simulink model "car_sim"  (R2022a)
settings: Solver=FixedStepAuto  StartTime=0.0  StopTime=40  FixedStep=0.001  RelTol=1e-3
InitFcn:
  | init_car_dynamic
StopFcn:
  | plot_traj_results
undefined symbols (not defined in the file or in its folder): ctrl_K, ctrl_K_lqi, ModelParams, my_traj, track, trackWidth, traj, vx
libraries: slpidlib x3
settings Model: Creator=Manny  LastModifiedBy=zqsyx
settings SolverCC: AlgebraicLoopSolver=LineSearch
settings DebuggingCC: UnconnectedInputMsg=warning  UnconnectedOutputMsg=warning  UnconnectedLineMsg=warning  SFMachineParentedDataDiag=warning
settings RTWCC: DLArmComputeVersion=19.05

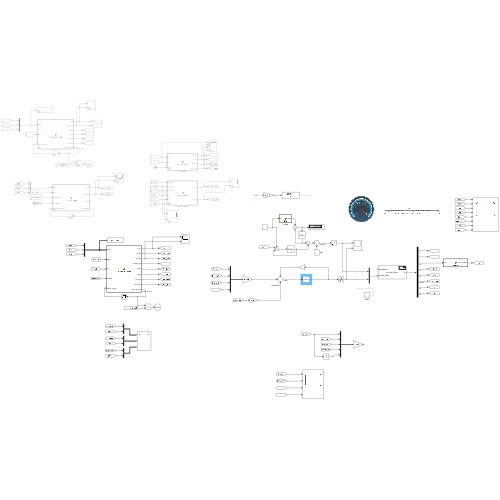
[thumbnail: Simulink's stored preview of the top-level diagram]
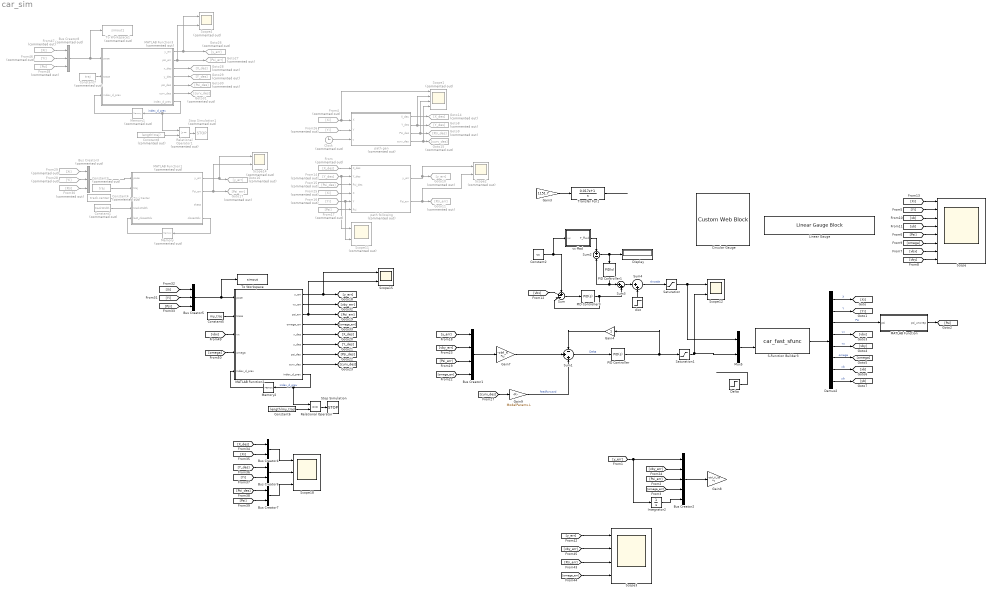
== system car_sim ==
  Bus Creator1 : BusCreator  Inputs=4
  Bus Creator2 : BusCreator  Inputs=5
  Bus Creator3 : BusCreator  Commented=on  Inputs=3
  Bus Creator4 : BusCreator  Inputs=2
  Bus Creator5 : BusCreator  Inputs=3
  Bus Creator6 : BusCreator  Inputs=2
  Bus Creator7 : BusCreator  Inputs=2
  Bus Creator8 : BusCreator  Commented=on  Inputs=3
  Circular Gauge : CustomWebBlock  LabelPosition=Hide  ShowInitialText=on  Configuration="{\"components\":[{\"name\":\"CircularScaleComponent\",\"settings\":{\"bounds\":{\"max\":1,\"min\":0,\"tickInterval\":\"auto\"},\"direction\":\"cw\",\"flipLimits\":0,\"innerRadius\":0.75,\"internalTickHeightScaleFactor\":1,\"labelColor\":[255,252,199],\"labelFont\":{\"font\":\"Arial\",\"fontSize\":12},\"labelTransparency\":1,\"minorTickHeightScaleFactor\":0.2,\"needleImage\":{\"size\":[1890,567],\"src\":\"data:image\\/svg+xml;base64,PD94bWwgdmVyc2lvbj0iMS4wIiBlbmNvZGluZz0iVVRGLTgiIHN0YW5kYWxvbmU9Im5vIj8+CjxzdmcKICAgeG1sbnM6ZGM9Imh0dHA6Ly9wdXJsLm9yZy9kYy9lbGVtZW50cy8xLjEvIgogICB4bWxuczpjYz0iaHR0cDovL2NyZWF0aXZlY29tbW9ucy5vcmcvbnMjIgogICB4bWxuczpyZGY9Imh0dHA6Ly93d3cudzMub3JnLzE5OTkvMDIvMjItcmRmLXN5bnRheC1ucyMiCiAgIHhtbG5zOnN2Zz0iaHR0cDovL3d3dy53My5vcmcvMjAwMC9zdmciCiAgIHhtbG5zPSJodHRwOi8vd3d3LnczLm9yZy8yMDAwL3N2ZyIKICAgeG1sbnM6 ...(+4096 chars)\"},\"needleOffset\":[0.1610917094974375,0],\"needleOrientation\":-45,\"needleRotation\":180.59702388394928,\"needleSize\":{\"height\":0.13032601008944536,\"width\":0.416859542883425},\"outerRadius\":0.9,\"position\":[0.06486742424242424,0.05627705627705628,0.8917748917748918,0.8787878787878788],\"scaleAngle\":270,\"scaleAngleOffset\":135,\"scaleColors\":[{\"color\":[0,114,189],\"max\":0.8,\"min\":0},{\"color\":[217,83,25],\"max\":1,\"min\":0.81}],\"scaleColorsSize\":0.2,\"scalePosition\":[0,0,1,1],\"showLabels\":1,\"showMinorTicks\":1,\"showSpanLine\":1,\"showTicks\":1,\"tickColor\":[255,255,200],\"tickTransparency\":1,\"valueBarColor\":[0,114,189],\"valueBarPosition\":[0,0,1,1],\"valueBarSize\":0.2,\"valueBarTransparency\":1}},{\"name\":\"BackgroundImageComponent\",\"settings\":{\"image\":{\"size\":[500,500],\"src\":\"data:image\\/svg+xml;base64,PD94bWwgdmVyc2lvbj0iMS4wIiBlbmNvZGluZz0iVVRGLTgiIHN0YW5kYWxvbmU9Im5vIj8+CjxzdmcKICAgeG1sbnM6ZGM9Imh0dHA6Ly9wdXJsLm9yZy9kYy9lbGVtZW50cy8xLjEvIgogICB4bWxuczpjYz0iaHR0cDovL2NyZWF0aXZlY29tbW9ucy5vcmcvbnMjIgogICB4bWxuczpyZGY9Imh0dHA6Ly93d3cudzMub3JnLzE5OTkvMDIvMjItcmRmLXN5bnRheC1ucyMiCiAgIHhtbG5zOnN2Zz0iaHR0cDovL3d3dy53My5vcmcvMjAwMC9zdmciCiAgIHhtbG5zPSJodHRwOi8vd3d3LnczLm9yZy8yMDAwL3N2ZyIKICAgeG1sbnM6 ...(+9964 chars)\"},\"position\":[0,0,1,1],\"scaleMode\":\"0\"}},{\"name\":\"ForegroundImageComponent\",\"settings\":{\"image\":{\"size\":[0,0],\"src\":\"default\",\"srcOrientation\":[]},\"isForeground\":1,\"position\":[0,0,1,1],\"scaleMode\":\"0\"}}],\"settings\":{\"BindingType\":\"signal\",\"aspectRatio\":1.0330578512396693,\"direction\":\"cw\",\"fixedAspectRatio\":\"on\",\"flipLimits\":0,\"orientation\":\"horizontal\"},\"type\":\"CircularGauge\"}"
  Clock : Clock  Commented=on
  Constant1 : Constant  Commented=on  Value=trackWidth
  Constant2 : Constant  Value=vx
  Constant3 : Constant  Commented=on  Value=traj  VectorParams1D=off  OutDataTypeStr=Bus: traj_bus
  Constant4 : Constant  Commented=on  Value=track.center
  Constant5 : Constant  Value=my_traj
  Constant6 : Constant  Value=length(my_traj)
  Constant7 : Constant  Commented=on  Value=traj
  Constant8 : Constant  Commented=on  Value=length(traj)
  Delta : Step  Time=5  After=0.05  SampleTime=0
  Demux2 : Demux  Outputs=8
  Display : Display
  From : From  Commented=on  GotoTag=X_des
  From14 : From  Commented=on  GotoTag=Y_des
  From15 : From  Commented=on  GotoTag=Psi_des
  From{16,26,28,46} (4 alike) : From  Commented=on  GotoTag=Yi
  From17 : From  Commented=on  GotoTag=Psi
  From{4,25,29,47} (4 alike) : From  Commented=on  GotoTag=Xi
  From30 : From  Commented=on  GotoTag=Psi
  From48 : From  Commented=on  GotoTag=Psi
  Gain3 : Gain  Gain=1151.7
  Gain4 : Gain
  Gain7 : Gain  Gain=-ctrl_K  Multiplication=Matrix(K*u) (u vector)
  Gain8 : Gain  Gain=-ctrl_K_lqi  Multiplication=Matrix(K*u) (u vector)
  Gain9 : Gain  Gain=ModelParams.L
  Goto10 : Goto  Commented=on  GotoTag=y_err
  Goto11 : Goto  Commented=on  GotoTag=Psi_err
  Goto14 : Goto  Commented=on  GotoTag=X_des
  Goto15 : Goto  Commented=on  GotoTag=curv_des
  Goto16 : Goto  Commented=on  GotoTag=y_err
  Goto17 : Goto  Commented=on  GotoTag=Psi_err
  Goto26 : Goto  Commented=on  GotoTag=y_err
  Goto27 : Goto  Commented=on  GotoTag=Psi_err
  Goto28 : Goto  Commented=on  GotoTag=X_des
  Goto29 : Goto  Commented=on  GotoTag=Y_des
  Goto30 : Goto  Commented=on  GotoTag=Psi_des
  Goto31 : Goto  Commented=on  GotoTag=curv_des
  Goto8 : Goto  Commented=on  GotoTag=Y_des
  Goto9 : Goto  Commented=on  GotoTag=Psi_des
  Integrator2 : Integrator
  Linear Gauge : LinearGaugeBlock  ScaleMin=-1.5  ScaleMax=1.5
  MATLAB Function : MATLAB Function  TreatAsAtomicUnit=on
  MATLAB Function1 : MATLAB Function  Commented=on  TreatAsAtomicUnit=on
  MATLAB Function2 : MATLAB Function  TreatAsAtomicUnit=on
  MATLAB Function3 : MATLAB Function  Commented=on  TreatAsAtomicUnit=on
  Memory : Memory  Commented=on
  Memory1 : Memory  Commented=on
  Memory2 : Memory
  Mux5 : Mux  Inputs=2
  PID Controller : slpidlib/PID Controller  Controller=PID  Form=Parallel  TimeDomain=Continuous-time  UseExternalTs=off  SampleTime=-1  IntegratorMethod=Forward Euler  FilterMethod=Forward Euler  ControllerParametersSource=internal  P=0.001  I=1.5  UseKiTs=off  D=1.8  N=100  UseFilter=on  TunerSelectOption=Transfer Function Based (PID Tuner App)  InitialConditionSource=internal  InitialConditionForIntegrator=0  InitialConditionForFilter=0  DifferentiatorICPrevScaledInput=0  ExternalReset=none  TrackingMode=off  Kt=0.5  LimitOutput=off  SatLimitsSource=internal  UpperSaturationLimit=inf  LowerSaturationLimit=-inf  LinearizeAsGain=on  AntiWindupMode=none  Kb=1  POutMin=[]  POutMax=[]  IOutMin=[]  IOutMax=[]  DOutMin=[]  DOutMax=[]  NOutMin=[]  NOutMax=[]  SumOutMin=[]  SumOutMax=[]  SaturationOutMin=[]  SaturationOutMax=[]  PParamMin=[]  PParamMax=[]  IParamMin=[]  IParamMax=[]  DParamMin=[]  DParamMax=[]  NParamMin=[]  NParamMax=[]  KbParamMin=[]  KbParamMax=[]  KtParamMin=[]  KtParamMax=[]  KbOutMin=[]  KbOutMax=[]  KtOutMin=[]  KtOutMax=[]  IntegratorOutMin=[]  IntegratorOutMax=[]  FilterOutMin=[]  FilterOutMax=[]  SumI1OutMin=[]  SumI1OutMax=[]  SumI2OutMin=[]  SumI2OutMax=[]  SumI3OutMin=[]  SumI3OutMax=[]  SumI4OutMin=[]  SumI4OutMax=[]  SumDOutMin=[]  SumDOutMax=[]  DifferentiatorOutMin=[]  DifferentiatorOutMax=[]  FilterDiffOutCoefMin=[]  FilterDiffOutCoefMax=[]  ReciprocalOutMin=[]  ReciprocalOutMax=[]  SumDenOutMin=[]  SumDenOutMax=[]  SumNumOutMin=[]  SumNumOutMax=[]  DivideOutMin=[]  DivideOutMax=[]  UdiffTsProdOutMin=[]  UdiffTsProdOutMax=[]  NTsProdOutMin=[]  NTsProdOutMax=[]  UintegralTsProdOutMin=[]  UintegralTsProdOutMax=[]  UngainTsProdOutMin=[]  UngainTsProdOutMax=[]  IntegratorContinuousStateAttributes=''  IntegratorStateMustResolveToSignalObject=off  IntegratorRTWStateStorageClass=Auto  FilterContinuousStateAttributes=''  FilterStateMustResolveToSignalObject=off  FilterRTWStateStorageClass=Auto  ParallelPVariant=InternalParameters  IdealPVariant=Disabled  IVariant=InternalParameters  DVariant=InternalParameters  IntegratorVariant=Continuous  SatVariant=Disabled  AWVariant=Passthrough  PCopyVariant=Disabled  TRVariant=Disabled  FdbkBlocksVariant=Forward  IdealPFdbkVariant=Disabled  SatFdbkVariant=Disabled  DerivativeFilterVariant=ContFilter  NVariant=InternalParameters  NCopyVariant=Disabled  FilterICVariant=InternalICsFilter  IntegratorICVariant=InternalICs  ExternalResetVariant=Disabled  TRSumVariant=Passthrough  SumFdbkVariant=Disabled  SumVariant=Sum_PID  TsampFilterVariant=InternalTs  TsampNgainVariant=Passthrough  TsampIntegralVariant=Passthrough  ExternalSaturationOutDataTypeStr=Inherit: Same as second input  aMode=0
  PID Controller1 : slpidlib/PID Controller  Controller=PID  Form=Parallel  TimeDomain=Continuous-time  UseExternalTs=off  SampleTime=-1  IntegratorMethod=Forward Euler  FilterMethod=Forward Euler  ControllerParametersSource=internal  P=0.001  I=1.5  UseKiTs=off  D=1.8  N=100  UseFilter=on  TunerSelectOption=Transfer Function Based (PID Tuner App)  InitialConditionSource=internal  InitialConditionForIntegrator=0  InitialConditionForFilter=0  DifferentiatorICPrevScaledInput=0  ExternalReset=none  TrackingMode=off  Kt=0.5  LimitOutput=off  SatLimitsSource=internal  UpperSaturationLimit=inf  LowerSaturationLimit=-inf  LinearizeAsGain=on  AntiWindupMode=none  Kb=1  POutMin=[]  POutMax=[]  IOutMin=[]  IOutMax=[]  DOutMin=[]  DOutMax=[]  NOutMin=[]  NOutMax=[]  SumOutMin=[]  SumOutMax=[]  SaturationOutMin=[]  SaturationOutMax=[]  PParamMin=[]  PParamMax=[]  IParamMin=[]  IParamMax=[]  DParamMin=[]  DParamMax=[]  NParamMin=[]  NParamMax=[]  KbParamMin=[]  KbParamMax=[]  KtParamMin=[]  KtParamMax=[]  KbOutMin=[]  KbOutMax=[]  KtOutMin=[]  KtOutMax=[]  IntegratorOutMin=[]  IntegratorOutMax=[]  FilterOutMin=[]  FilterOutMax=[]  SumI1OutMin=[]  SumI1OutMax=[]  SumI2OutMin=[]  SumI2OutMax=[]  SumI3OutMin=[]  SumI3OutMax=[]  SumI4OutMin=[]  SumI4OutMax=[]  SumDOutMin=[]  SumDOutMax=[]  DifferentiatorOutMin=[]  DifferentiatorOutMax=[]  FilterDiffOutCoefMin=[]  FilterDiffOutCoefMax=[]  ReciprocalOutMin=[]  ReciprocalOutMax=[]  SumDenOutMin=[]  SumDenOutMax=[]  SumNumOutMin=[]  SumNumOutMax=[]  DivideOutMin=[]  DivideOutMax=[]  UdiffTsProdOutMin=[]  UdiffTsProdOutMax=[]  NTsProdOutMin=[]  NTsProdOutMax=[]  UintegralTsProdOutMin=[]  UintegralTsProdOutMax=[]  UngainTsProdOutMin=[]  UngainTsProdOutMax=[]  IntegratorContinuousStateAttributes=''  IntegratorStateMustResolveToSignalObject=off  IntegratorRTWStateStorageClass=Auto  FilterContinuousStateAttributes=''  FilterStateMustResolveToSignalObject=off  FilterRTWStateStorageClass=Auto  ParallelPVariant=InternalParameters  IdealPVariant=Disabled  IVariant=InternalParameters  DVariant=InternalParameters  IntegratorVariant=Continuous  SatVariant=Disabled  AWVariant=Passthrough  PCopyVariant=Disabled  TRVariant=Disabled  FdbkBlocksVariant=Forward  IdealPFdbkVariant=Disabled  SatFdbkVariant=Disabled  DerivativeFilterVariant=ContFilter  NVariant=InternalParameters  NCopyVariant=Disabled  FilterICVariant=InternalICsFilter  IntegratorICVariant=InternalICs  ExternalResetVariant=Disabled  TRSumVariant=Passthrough  SumFdbkVariant=Disabled  SumVariant=Sum_PID  TsampFilterVariant=InternalTs  TsampNgainVariant=Passthrough  TsampIntegralVariant=Passthrough  ExternalSaturationOutDataTypeStr=Inherit: Same as second input  aMode=0
  PID Controller3 : slpidlib/PID Controller  Controller=PID  Form=Parallel  TimeDomain=Continuous-time  UseExternalTs=off  SampleTime=-1  IntegratorMethod=Forward Euler  FilterMethod=Forward Euler  ControllerParametersSource=internal  P=0.001  I=1.5  UseKiTs=off  D=1.8  N=100  UseFilter=on  TunerSelectOption=Transfer Function Based (PID Tuner App)  InitialConditionSource=internal  InitialConditionForIntegrator=0  InitialConditionForFilter=0  DifferentiatorICPrevScaledInput=0  ExternalReset=none  TrackingMode=off  Kt=0.5  LimitOutput=off  SatLimitsSource=internal  UpperSaturationLimit=inf  LowerSaturationLimit=-inf  LinearizeAsGain=on  AntiWindupMode=none  Kb=1  POutMin=[]  POutMax=[]  IOutMin=[]  IOutMax=[]  DOutMin=[]  DOutMax=[]  NOutMin=[]  NOutMax=[]  SumOutMin=[]  SumOutMax=[]  SaturationOutMin=[]  SaturationOutMax=[]  PParamMin=[]  PParamMax=[]  IParamMin=[]  IParamMax=[]  DParamMin=[]  DParamMax=[]  NParamMin=[]  NParamMax=[]  KbParamMin=[]  KbParamMax=[]  KtParamMin=[]  KtParamMax=[]  KbOutMin=[]  KbOutMax=[]  KtOutMin=[]  KtOutMax=[]  IntegratorOutMin=[]  IntegratorOutMax=[]  FilterOutMin=[]  FilterOutMax=[]  SumI1OutMin=[]  SumI1OutMax=[]  SumI2OutMin=[]  SumI2OutMax=[]  SumI3OutMin=[]  SumI3OutMax=[]  SumI4OutMin=[]  SumI4OutMax=[]  SumDOutMin=[]  SumDOutMax=[]  DifferentiatorOutMin=[]  DifferentiatorOutMax=[]  FilterDiffOutCoefMin=[]  FilterDiffOutCoefMax=[]  ReciprocalOutMin=[]  ReciprocalOutMax=[]  SumDenOutMin=[]  SumDenOutMax=[]  SumNumOutMin=[]  SumNumOutMax=[]  DivideOutMin=[]  DivideOutMax=[]  UdiffTsProdOutMin=[]  UdiffTsProdOutMax=[]  NTsProdOutMin=[]  NTsProdOutMax=[]  UintegralTsProdOutMin=[]  UintegralTsProdOutMax=[]  UngainTsProdOutMin=[]  UngainTsProdOutMax=[]  IntegratorContinuousStateAttributes=''  IntegratorStateMustResolveToSignalObject=off  IntegratorRTWStateStorageClass=Auto  FilterContinuousStateAttributes=''  FilterStateMustResolveToSignalObject=off  FilterRTWStateStorageClass=Auto  ParallelPVariant=InternalParameters  IdealPVariant=Disabled  IVariant=InternalParameters  DVariant=InternalParameters  IntegratorVariant=Continuous  SatVariant=Disabled  AWVariant=Passthrough  PCopyVariant=Disabled  TRVariant=Disabled  FdbkBlocksVariant=Forward  IdealPFdbkVariant=Disabled  SatFdbkVariant=Disabled  DerivativeFilterVariant=ContFilter  NVariant=InternalParameters  NCopyVariant=Disabled  FilterICVariant=InternalICsFilter  IntegratorICVariant=InternalICs  ExternalResetVariant=Disabled  TRSumVariant=Passthrough  SumFdbkVariant=Disabled  SumVariant=Sum_PID  TsampFilterVariant=InternalTs  TsampNgainVariant=Passthrough  TsampIntegralVariant=Passthrough  ExternalSaturationOutDataTypeStr=Inherit: Same as second input  aMode=0
  Relational Operator : RelationalOperator  OutDataTypeStr=boolean  RndMeth=Simplest  InputSameDT=off
  Relational Operator1 : RelationalOperator  Commented=on  OutDataTypeStr=boolean  RndMeth=Simplest  InputSameDT=off
  S-Function Builder3 : S-Function  FunctionName=car_fast_sfunc  SFunctionModules=car_fast_sfunc_wrapper  SFunctionDeploymentMode=off  EnableBusSupport=off  mask(S-Function Builder){}
      mask help: Simulink:masks:SFunctionBuilder_MD
      mask init:
      | val = [[.9  0.75 0.75 1 1 .9 .9 1]',[1 1 0.75 0.75 .9 .9 1 .9]'];try , sys = get_param(gcb,'SfunBuilderFcnName');if isempty(sys), sys = get_param(gcb,'FunctionName'); end,catch, sys = get_param(gcb,'FunctionName'); end
      settings: CopyFcn=set_param(gcbh,'LinkStatus','none')  OpenFcn=sfunctionwizard(gcbh)
      mask Display:
      | plot(val(:,1),val(:,2))
      | disp(sys)
      | port_label('input',1,'disturbance')
      | port_label('input',2,'throttle_delta')
      | port_label('output',1,'y0')
  Saturation : Saturate  UpperLimit=1  LowerLimit=0
  Saturation1 : Saturate  UpperLimit=pi/3  LowerLimit=-pi/3
  Scope : Scope  NumInputPorts=8
  Scope1 : Scope  Commented=on  NumInputPorts=4
  Scope{2,4,11,14} (4 alike) : Scope  Commented=on  NumInputPorts=2
  Scope12 : Scope  NumInputPorts=2
  Scope15 : Scope  NumInputPorts=2
  Scope18 : Scope  NumInputPorts=3
  Scope3 : Scope  NumInputPorts=4
  Stop Simulation : Stop
  Stop Simulation1 : Stop  Commented=on
  Sum : Sum  Inputs=+--|
  Sum1 : Sum  Inputs=-|+|+
  Sum2 : Sum  Inputs=+|-
  Sum3 : Sum  Inputs=|++
  Sum4 : Sum  Inputs=|++
  To Workspace : ToWorkspace  VariableName=simout  SaveFormat=Timeseries  SampleTime=-1
  To Workspace1 : ToWorkspace  Commented=on  VariableName=simout1  SaveFormat=Timeseries  SampleTime=-1
  Transfer Fcn1 : TransferFcn  Numerator=[0.017 1]  Denominator=[1 0]
  dist : Step  After=-0.05  SampleTime=0
  path following : MATLAB Function  Commented=on  TreatAsAtomicUnit=on
  path gen : MATLAB Function  Commented=on  TreatAsAtomicUnit=on
  vx ffwd : MATLAB Function  TreatAsAtomicUnit=on
  wires:
  S-Function Builder3/1 -> Demux2/1
  Mux5/1 -> S-Function Builder3/2
  Demux2/1 -> [Xi]  "X"
  Demux2/2 -> [Yi]  "Y"
  Demux2/3 -> MATLAB Function/1(psi)  "Psi"
  Demux2/4 -> [vbx]  "vx"
  Demux2/5 -> [vby]  "vy"
  Demux2/6 -> [omega]  "omega"
  Demux2/7 -> [xb]  "xb"
  Demux2/8 -> [yb]  "yb"
  [vby_err] -> Bus Creator1/2
  [omega_err] -> Bus Creator1/4
  Bus Creator1/1 -> Gain7/1
  [Xi] -> Scope/1
  [Yi] -> Scope/2
  [xb] -> Scope/3
  [yb] -> Scope/4
  [Psi] -> Scope/5
  [vbx] -> Scope/7
  [vby] -> Scope/8
  [omega] -> Scope/6
  [y_err] -> Bus Creator1/1
  [Psi_err] -> Bus Creator1/3
  From4/1 -> Scope1/1, path gen/1(X)
  path gen/3(Psi_des) -> Scope1/3, Goto9/1
  path gen/2(Y_des) -> Goto8/1, Scope1/2
  From14/1 -> Scope11/1, path following/2(Y_des)
  From15/1 -> path following/3(Psi_des)
  From16/1 -> Scope11/2, path following/5(Y)
  From17/1 -> path following/6(Psi)
  path following/1(y_err) -> Scope2/1, Goto10/1
  path following/2(Psi_err) -> Scope2/2, Goto11/1
  Delta/1 -> ?
  [y_err] -> Integrator2/1, Bus Creator2/1
  Bus Creator2/1 -> Gain8/1
  [omega_err] -> Bus Creator2/4
  [vby_err] -> Bus Creator2/2
  Integrator2/1 -> Bus Creator2/5
  Clock/1 -> path gen/3(t)
  Sum1/1 -> PID Controller/1  "Delta"
  Gain9/1 -> Sum1/3  "feedforward"
  From25/1 -> path following/4(X)
  path gen/1(X_des) -> Goto14/1
  From/1 -> path following/1(X_des)
  From26/1 -> path gen/2(Y)
  Saturation/1 -> Mux5/1, Scope12/1
  Saturation1/1 -> Mux5/2, Scope12/2
  path gen/4(curv_des) -> Scope1/4, Goto15/1
  [curv_des] -> Gain9/1
  MATLAB Function/1(psi_unwrap) -> [Psi]
  MATLAB Function1/4(closestIdx) -> Memory/1
  Memory/1 -> MATLAB Function1/5(last_closestIdx)
  Constant1/1 -> MATLAB Function1/4(trackWidth)
  Bus Creator3/1 -> MATLAB Function1/1(pose)
  From29/1 -> Bus Creator3/1
  From28/1 -> Bus Creator3/2
  From30/1 -> Bus Creator3/3
  MATLAB Function1/1(y_err) -> Goto16/1, Scope14/1
  MATLAB Function1/2(Psi_err) -> Scope14/2, Goto17/1
  Constant3/1 -> MATLAB Function1/2(traj)
  Constant4/1 -> MATLAB Function1/3(TrackCenter)
  [Yi] -> Bus Creator5/2
  [Xi] -> Bus Creator5/1
  Bus Creator5/1 -> To Workspace/1, MATLAB Function2/1(pose)
  [Psi] -> Bus Creator5/3
  MATLAB Function2/5(x_des) -> [X_des]
  MATLAB Function2/7(psi_des) -> [Psi_des]
  MATLAB Function2/6(y_des) -> [Y_des]
  [X_des] -> Bus Creator4/1
  [Xi] -> Bus Creator4/2
  [Yi] -> Bus Creator6/2
  [Y_des] -> Bus Creator6/1
  [Psi_des] -> Bus Creator7/1
  [Psi] -> Bus Creator7/2
  Bus Creator4/1 -> Scope18/1
  Bus Creator6/1 -> Scope18/2
  Bus Creator7/1 -> Scope18/3
  MATLAB Function2/8(curv_des) -> [curv_des]
  MATLAB Function2/9(index_d_prev) -> Relational Operator/1, Memory2/1  "index_d_prev"
  Memory2/1 -> MATLAB Function2/5("index_d_prev ")
  MATLAB Function2/1(y_err) -> [y_err], Scope15/1
  MATLAB Function2/3(psi_err) -> [Psi_err], Scope15/2
  Relational Operator/1 -> Stop Simulation/1
  Constant6/1 -> Relational Operator/2
  [y_err] -> Scope3/1
  [vby_err] -> Scope3/2
  [Psi_err] -> Scope3/3
  [omega_err] -> Scope3/4
  ? -> Gain3/1
  Gain3/1 -> Transfer Fcn1/1
  Transfer Fcn1/1 -> ?
  Constant8/1 -> Relational Operator1/2
  Relational Operator1/1 -> Stop Simulation1/1
  MATLAB Function3/2(psi_err) -> Scope4/2, Goto27/1
  MATLAB Function3/1(y_err) -> Goto26/1, Scope4/1
  Memory1/1 -> MATLAB Function3/3("index_d_prev ")
  MATLAB Function3/7(index_d_prev) -> Memory1/1, Relational Operator1/1  "index_d_prev"
  MATLAB Function3/6(curv_des) -> Goto31/1
  MATLAB Function3/4(y_des) -> Goto29/1
  MATLAB Function3/5(psi_des) -> Goto30/1
  MATLAB Function3/3(x_des) -> Goto28/1
  From48/1 -> Bus Creator8/3
  Constant7/1 -> MATLAB Function3/2(trace)
  Bus Creator8/1 -> MATLAB Function3/1(pose), To Workspace1/1
  From47/1 -> Bus Creator8/1
  From46/1 -> Bus Creator8/2
  [vbx] -> MATLAB Function2/3(vx)
  [omega] -> MATLAB Function2/4(omega)
  MATLAB Function2/4(omega_err) -> [omega_err]
  MATLAB Function2/2(vy_err) -> [vby_err]
  Constant5/1 -> MATLAB Function2/2(trace)
  [Psi_err] -> Bus Creator2/3
  Gain7/1 -> Sum1/2
  PID Controller/1 -> Gain4/1, Saturation1/1
  dist/1 -> Sum4/2
  Sum4/1 -> Saturation/1  "throttle"
  Gain4/1 -> Sum1/1
  Sum3/1 -> Sum4/1
  Constant2/1 -> Sum/1, vx ffwd/1(vx)
  PID Controller1/1 -> Sum2/2, Sum3/1
  PID Controller3/1 -> Sum/3, Sum3/2
  [vbx] -> Sum/2
  vx ffwd/1(T_ffwd) -> Sum2/1
  Sum2/1 -> PID Controller1/1, Display/1
  Sum/1 -> PID Controller3/1

== matlab function car_sim/MATLAB Function3 ==
  data: y_err output; psi_err output; pose input; trace input; x_des output; y_des output; psi_des output; curv_des output; index_d_prev input; index_d_prev output
function [y_err,psi_err,x_des,y_des,psi_des,curv_des, index_d_prev]=cal_nearest_index(pose, trace, index_d_prev)

traj_x=trace(1,:);      %给定x坐标
traj_y=trace(2,:);      %给定y坐标
traj_psi=trace(3,:);    %给定航向角Psi
traj_k=trace(4,:);      %曲率

x = pose(1);
y = pose(2);
psi = pose(3);

dx=x*ones(1,length(traj_x))-traj_x;
dy=y*ones(1,length(traj_y))-traj_y;

% find the nearest index
d=dx.^2+dy.^2;
[mini_d,index_d]=min(d);

% go forward
if index_d <= index_d_prev
    index_d = index_d_prev;
end

index_d_prev = index_d;
dis=sqrt(mini_d);

% current position point to designed positon
dx1=traj_x(index_d)-x;
dy1=traj_y(index_d)-y;

% yaw vector [cos(psi_des) sin(psi_des)]
axis = cross([dx1 dy1 1], [cos(traj_psi(index_d)) sin(traj_psi(index_d)) 1]);

if axis(3)<0
    dis=-dis;
end

psi_des = pi_2_pi(traj_psi(index_d));
x_des = traj_x(index_d);
y_des = traj_y(index_d);
curv_des = traj_k(index_d);

psi_err = psi - psi_des;
psi_err = pi_2_pi(psi_err);
y_err = dis;

% TODO: add the psi_dot and y_dot command

end

function angle=pi_2_pi(angle)
if angle > pi
    angle=angle-2*pi;
elseif angle < -pi
    angle=angle+2*pi;
end
end

== matlab function car_sim/path following ==
  data: X_des input; y_err output; Psi_err output; Y_des input; Psi_des input; X input; Y input; Psi input
function [y_err,Psi_err] = path_following(X_des,Y_des,Psi_des,X,Y,Psi)


y_err = (Y-Y_des)/cos(Psi)*2;

% y_err = -(X-X_des)/sin(Psi);

Psi_err = (Psi - Psi_des)*2;

== matlab function car_sim/path gen ==
  data: X_des output; Y_des output; X input; Y input; Psi_des output; t input; curv_des output
function [X_des,Y_des,Psi_des,curv_des] = path_generator(X,Y,t)

path_omega = 0.01+0.001*t;
X_des=X;
Y_des=sin(path_omega*X);
Psi_des = atan(path_omega*cos(path_omega*X));

% TODO: add curvature: https://en.wikipedia.org/wiki/Curvature
% curv_des = (-path_omega^2*sin(path_omega*X))/(1+(path_omega*cos(path_omega*X))^2)^1.5;

path_omega = 0.3;
X_des = 10*sin(path_omega*t);
Y_des = 10-10*cos(path_omega*t);
Psi_des = atan2(10*path_omega*cos(path_omega*t), 10*path_omega*sin(path_omega*t));
vx_des = 10*path_omega;

== matlab function car_sim/MATLAB Function ==
  data: psi input; psi_unwrap output
function psi_unwrap = unwrap(psi)

if ( psi > pi)
    psi = psi - 2*pi;
end

if( psi <= -pi)
    psi = psi + 2*pi;
end

psi_unwrap = psi;

== matlab function car_sim/MATLAB Function1 ==
  data: y_err output; Psi_err output; pose input; traj input; TrackCenter input; theta output; trackWidth input; last_closestIdx input; closestIdx output
function [y_err, Psi_err, theta, closestIdx] = path_following(pose, traj, TrackCenter, trackWidth, last_closestIdx)
%FINDTHETA returns theta, the index of the point on the centerline which is the
%closest to the current position

%the algorithm first performs a local search around a guess where the
%closest point on the center line is if the error is too big (more than
%half the track width) a global search is performed.

%then the projection is computed using the inner product and assuming the
%track is picewise affine

traj.ppx.form = 'pp';
traj.ppy.form = 'pp';
traj.dppx.form = 'pp';
traj.dppy.form = 'pp';
traj.ddppx.form = 'pp';
traj.ddppy.form = 'pp';

traj_breaks = traj.ppx.breaks;
posX = pose(1);
posY = pose(2);
Psi = pose(3);
TrackX = TrackCenter(1,:);
TrackY = TrackCenter(2,:);
trackCenterline = TrackCenter;
N_Track = length(TrackX);

% length of local search region
N_searchRegion = 26;
searchRegion = zeros(1,N_searchRegion);
% determin index which are investigated
k = 1;
for i = last_closestIdx-5:last_closestIdx+20
    searchRegion(k) = i;
    k = k+1;
end
% wrapping if necessary
if last_closestIdx > N_Track - 20 || last_closestIdx <= 5
    i = find(searchRegion < 1);
    k = find(searchRegion > N_Track);
    searchRegion(i) = N_Track+searchRegion(i);
    searchRegion(k) = searchRegion(k)-N_Track;
end

% compute squared distance to the current location
TrackXsmall = TrackX(searchRegion);
TrackYsmall = TrackY(searchRegion);
distanceX = TrackXsmall - posX*ones(1,N_searchRegion);
distanceY = TrackYsmall - posY*ones(1,N_searchRegion);

squared_distance_array   = distanceX.^2 + distanceY.^2;
% find closest point
[e , minIndex] = min(squared_distance_array);
minIndex = searchRegion(minIndex);

% if distance is to large perform global search with respect to track width
if sqrt(e) > (trackWidth*1.25)/2
    distanceX2 = TrackX - posX*ones(1,N_Track);
    distanceY2 = TrackY - posY*ones(1,N_Track);

    squared_distance_array2   = distanceX2.^2 + distanceY2.^2;

    [e , minIndex] = min(squared_distance_array2);
end

% circular edge conditions
if minIndex == 1
    nextIdx = 2;
    prevIdx = N_Track;
elseif minIndex == N_Track
    nextIdx = 1;
    prevIdx = N_Track-1;
else
    nextIdx = minIndex + 1;
    prevIdx = minIndex - 1;
end


% compute theta based on inner product projection
closestIdx = minIndex;
cosinus = dot([posX;posY] - trackCenterline(:,minIndex), trackCenterline(:,prevIdx) - trackCenterline(:,minIndex));
if (cosinus > 0)
    minIndex2 = prevIdx;
else
    minIndex2 = minIndex;
    minIndex = nextIdx;
end


if e ~= 0
    cosinus = dot([posX;posY] - trackCenterline(:,minIndex2), trackCenterline(:,minIndex) - trackCenterline(:,minIndex2))/...
                 (norm([posX;posY] - trackCenterline(:,minIndex2))*norm(trackCenterline(:,minIndex) - trackCenterline(:,minIndex2)));
else
    cosinus = 0;
end
theta = traj_breaks(1,minIndex2);
theta = theta + cosinus*norm([posX;posY] - trackCenterline(:,minIndex2),2);

Psi_des = atan2(ppval(traj.dppy,theta),ppval(traj.dppx,theta));
X_des = ppval(traj.ppx,theta);
Y_des = ppval(traj.ppy,theta);
y_err = (Y-Y_des)/cos(Psi);
% y_err = -(X-X_des)/sin(Psi);
Psi_err = Psi - Psi_des;

return

== matlab function car_sim/MATLAB Function2 ==
  data: y_err output; vy_err output; psi_err output; omega_err output; pose input; trace input; vx input; omega input; x_des output; y_des output; psi_des output; curv_des output; index_d_prev input; index_d_prev output
function [y_err,vy_err,psi_err,omega_err,x_des,y_des,psi_des,curv_des, index_d_prev]=cal_nearest_index(pose,trace,vx, omega, index_d_prev)

traj_x=trace(1,:);      %给定x坐标
traj_y=trace(2,:);      %给定y坐标
traj_psi=trace(3,:);
traj_k=trace(4,:);      %曲率


x = pose(1);
y = pose(2);
psi = pose(3);

dx=x*ones(1,length(traj_x))-traj_x;
dy=y*ones(1,length(traj_y))-traj_y;

% find the nearest index
d=dx.^2+dy.^2;
[mini_d,index_d]=min(d);

% go forward
if index_d <= index_d_prev
    index_d = index_d_prev;
end

index_d_prev = index_d;
dis=sqrt(mini_d);

% current position point to designed positon
dx1=traj_x(index_d)-x;
dy1=traj_y(index_d)-y;

% yaw vector [cos(psi_des) sin(psi_des)]
axis = cross([dx1 dy1 1], [cos(traj_psi(index_d)) sin(traj_psi(index_d)) 1]);

if axis(3)<0
    dis=-dis;
end

psi_des = pi_2_pi(traj_psi(index_d));
x_des = traj_x(index_d);
y_des = traj_y(index_d);
curv_des = traj_k(index_d);

psi_err = psi - psi_des;
psi_err = pi_2_pi(psi_err);
y_err = dis;

% give a better vy_err and omega_err
% vy_err = vx*cos(psi_err);
% omega_des = vx*curv_des;
% omega_err = omega - omega_des;

vy_err = 1*y_err;
omega_err = 1*psi_err;

end

function angle=pi_2_pi(angle)
if angle > pi
    angle=angle-2*pi;
elseif angle < -pi
    angle=angle+2*pi;
end
end

== matlab function car_sim/vx ffwd ==
  data: vx input; T_ffwd output
function T_ffwd = fcn(vx)

m = 0.041;
g = 9.8;
Iz = 27.8e-6;
lf = 0.029;
lr = 0.033;
Cm1=0.287;
Cm2=0.0545;
Cr0=0.0218;
Cr2=0.00035;

Nf = m*g*lr/(lf+lr);
Nr = m*g*lf/(lf+lr);

T_ffwd = -(-Cr0*m*g-2*Cr2*vx^2)/(Cm1-Cm2*vx);
